simulink model "Part1_planarBicopter"  (R2020b)
settings: Solver=ode1  StartTime=0.0  StopTime=100  FixedStep=0.001  RelTol=1e-3
undefined symbols (not defined in the file or in its folder): Kd_alt, Kd_pos, Kd_roll, Kp_alt, Kp_pos, Kp_roll, noise, u_star, variaciones, wind, x_star
libraries: commchan3 x3
settings Model: Creator=rushik  LastModifiedBy=da_co
settings DataIOCC: SaveState=on

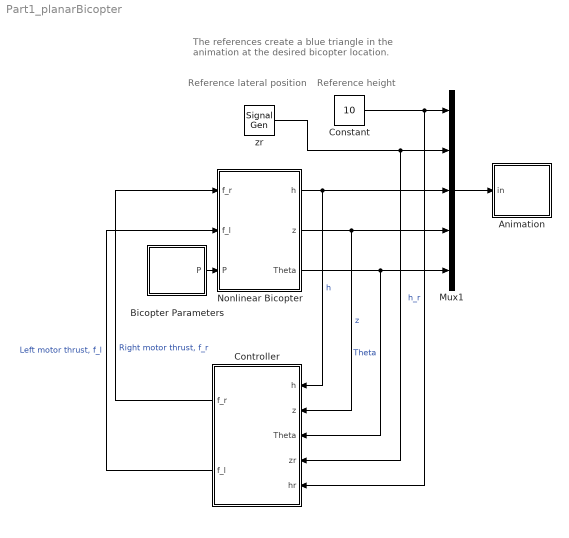
== system Part1_planarBicopter ==
  note: The references create a blue triangle in the
      | animation at the desired bicopter location.
  note: Reference height
  note: Reference lateral position
  Animation : Subsystem  mask(Pendulum plot){}
      mask help: Pendulum plot
      mask Help: Pendulum animation function using Handle graphics.
      mask Display: plot([-2 2],[10 10],[-2.5 -1.5],[10.5 10.5],[1.5 2.5],[10.5 10.5],0,0,0,20)
  Bicopter Parameters : Subsystem  mask{M=1, mRotor=0.25, J=0.0042, d=0.3, mu=0.1, g=9.81, x0=[0;0;0;0;0;0], noVar=noise, vWind=wind, distPercent=variaciones}
      mask prompts: M "Hub Mass"; mRotor "Motor Propeller Mass"; J "Hub Inertia"; d "Arm Length"; mu "Momentum Drag Coefficient"; g "Gravity"; x0 "Initial State"; noVar "Noise Variance"; vWind "Wind Velocity"; distPercent "Parameter Variation Percentage"
      mask TypeOptions M: Constant1/Value
      mask TypeOptions mRotor: Constant2/Value
      mask TypeOptions J: Constant3/Value
      mask TypeOptions d: Constant4/Value
      mask TypeOptions mu: Constant5/Value
      mask TypeOptions g: Constant6/Value
      mask TypeOptions x0: Constant7/Value
      mask TypeOptions noVar: Constant8/Value
      mask TypeOptions vWind: Constant10/Value
      mask TypeOptions distPercent: Constant9/Value
  Constant : Constant  Value=10
  Controller : Subsystem
  Mux1 : Mux  Inputs=5
  Nonlinear Bicopter : Subsystem
  zr : SignalGenerator  WaveForm=square  Amplitude=1.5  Frequency=0.05
  wires:
  Nonlinear Bicopter/1(h) -> Controller/1(h), Mux1/3  "h"
  Nonlinear Bicopter/2(z) -> Mux1/4, Controller/2(z)  "z"
  Nonlinear Bicopter/3(Theta) -> Mux1/5, Controller/3(Theta)  "Theta"
  Mux1/1 -> Animation/1(in)
  Bicopter Parameters/1(P) -> Nonlinear Bicopter/3(P)
  Controller/1(f_r) -> Nonlinear Bicopter/1(f_r)  "Right motor thrust, f_r"
  Controller/2(f_l) -> Nonlinear Bicopter/2(f_l)  "Left motor thrust, f_l"
  Constant/1 -> Controller/5(hr), Mux1/1  "h_r"
  zr/1 -> Controller/4(zr), Mux1/2

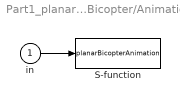
== system Part1_planarBicopter/Animation ==
  in : Inport
  S-function : S-Function  FunctionName=planarBicopterAnimation  SFunctionDeploymentMode=off  EnableBusSupport=off
      settings: DeleteFcn=pendan([],[],[],'DeleteBlock');
  wires:
  in/1 -> S-function/1

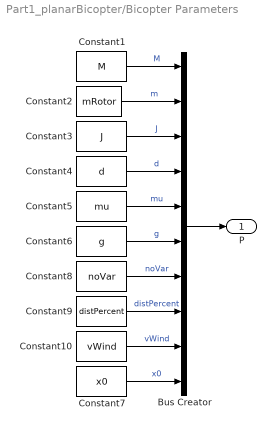
== system Part1_planarBicopter/Bicopter Parameters ==
  Bus Creator : BusCreator  Inputs=10
  Constant1 : Constant  Value=M
  Constant10 : Constant  Value=vWind  VectorParams1D=off
  Constant2 : Constant  Value=mRotor
  Constant3 : Constant  Value=J
  Constant4 : Constant  Value=d
  Constant5 : Constant  Value=mu
  Constant6 : Constant  Value=g
  Constant7 : Constant  Value=x0  VectorParams1D=off
  Constant8 : Constant  Value=noVar  VectorParams1D=off
  Constant9 : Constant  Value=distPercent  VectorParams1D=off
  P : Outport
  wires:
  Bus Creator/1 -> P/1
  Constant7/1 -> Bus Creator/10  "x0"
  Constant5/1 -> Bus Creator/5  "mu"
  Constant3/1 -> Bus Creator/3  "J"
  Constant2/1 -> Bus Creator/2  "m"
  Constant6/1 -> Bus Creator/6  "g"
  Constant4/1 -> Bus Creator/4  "d"
  Constant1/1 -> Bus Creator/1  "M"
  Constant8/1 -> Bus Creator/7  "noVar"
  Constant9/1 -> Bus Creator/8  "distPercent"
  Constant10/1 -> Bus Creator/9  "vWind"

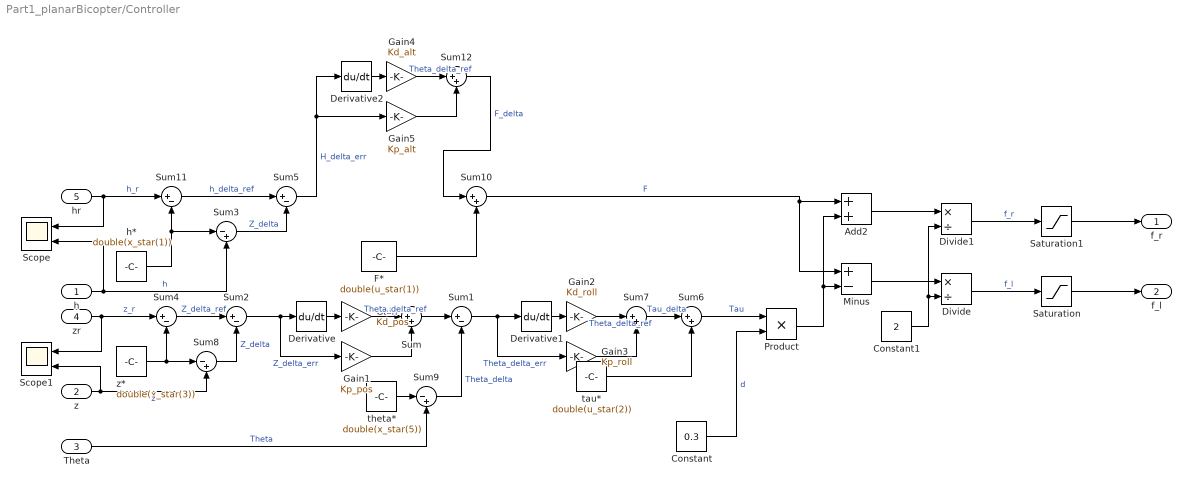
== system Part1_planarBicopter/Controller ==
  h : Inport
  z : Inport  Port=2
  Theta : Inport  Port=3
  zr : Inport  Port=4
  hr : Inport  Port=5
  Add2 : Sum
  Constant : Constant  Value=0.3
  Constant1 : Constant  Value=2
  Derivative : Derivative
  Derivative1 : Derivative
  Derivative2 : Derivative
  Divide : Product  Inputs=*/
  Divide1 : Product  Inputs=*/
  F* : Constant  Value=double(u_star(1))
  Gain : Gain  Gain=Kd_pos
  Gain1 : Gain  Gain=Kp_pos
  Gain2 : Gain  Gain=Kd_roll
  Gain3 : Gain  Gain=Kp_roll
  Gain4 : Gain  Gain=Kd_alt
  Gain5 : Gain  Gain=Kp_alt
  Minus : Sum  Inputs=+-
  Product : Product
  Saturation : Saturate  UpperLimit=10  LowerLimit=0
  Saturation1 : Saturate  UpperLimit=10  LowerLimit=0
  Scope : Scope  NumInputPorts=2
  Scope1 : Scope  NumInputPorts=2
  Sum{,6..7,10,12} (5 alike) : Sum  Inputs=|++
  Sum{1..2,4..5,11} (5 alike) : Sum  Inputs=|+-
  Sum3 : Sum  Inputs=|-+
  Sum8 : Sum  Inputs=|-+
  Sum9 : Sum  Inputs=|-+
  h* : Constant  Value=double(x_star(1))
  tau* : Constant  Value=double(u_star(2))
  theta* : Constant  Value=double(x_star(5))
  z* : Constant  Value=double(x_star(3))
  f_r : Outport
  f_l : Outport  Port=2
  wires:
  z/1 -> Scope1/2, Sum8/2  "z"
  Theta/1 -> Sum9/2  "Theta"
  zr/1 -> Sum4/1, Scope1/1  "z_r"
  Gain/1 -> Sum/1  "Theta_delta_ref"
  h/1 -> Scope/2, Sum3/2  "h"
  Minus/1 -> Divide/1
  Product/1 -> Minus/2, Add2/2
  Constant/1 -> Product/2  "d"
  Constant1/1 -> Divide1/2, Divide/2
  Add2/1 -> Divide1/1
  Sum10/1 -> Add2/1, Minus/1  "F"
  F*/1 -> Sum10/2
  Sum1/1 -> Gain3/1, Derivative1/1  "Theta_delta_err"
  Divide1/1 -> Saturation1/1  "f_r"
  Saturation1/1 -> f_r/1
  Divide/1 -> Saturation/1  "f_l"
  Saturation/1 -> f_l/1
  Sum12/1 -> Sum10/1  "F_delta"
  Sum2/1 -> Gain1/1, Derivative/1  "Z_delta_err"
  hr/1 -> Sum11/1, Scope/1  "h_r"
  Sum4/1 -> Sum2/1  "Z_delta_ref"
  z*/1 -> Sum8/1, Sum4/2
  theta*/1 -> Sum9/1
  Sum7/1 -> Sum6/1  "Tau_delta"
  tau*/1 -> Sum6/2
  Sum6/1 -> Product/1  "Tau"
  Sum8/1 -> Sum2/2  "Z_delta"
  Sum9/1 -> Sum1/2  "Theta_delta"
  Sum11/1 -> Sum5/1  "h_delta_ref"
  h*/1 -> Sum3/1, Sum11/2
  Sum3/1 -> Sum5/2  "Z_delta"
  Sum5/1 -> Gain5/1, Derivative2/1  "H_delta_err"
  Derivative/1 -> Gain/1
  Sum/1 -> Sum1/1
  Gain1/1 -> Sum/2
  Derivative1/1 -> Gain2/1
  Gain2/1 -> Sum7/1  "Theta_delta_ref"
  Gain3/1 -> Sum7/2
  Derivative2/1 -> Gain4/1
  Gain4/1 -> Sum12/1  "Theta_delta_ref"
  Gain5/1 -> Sum12/2

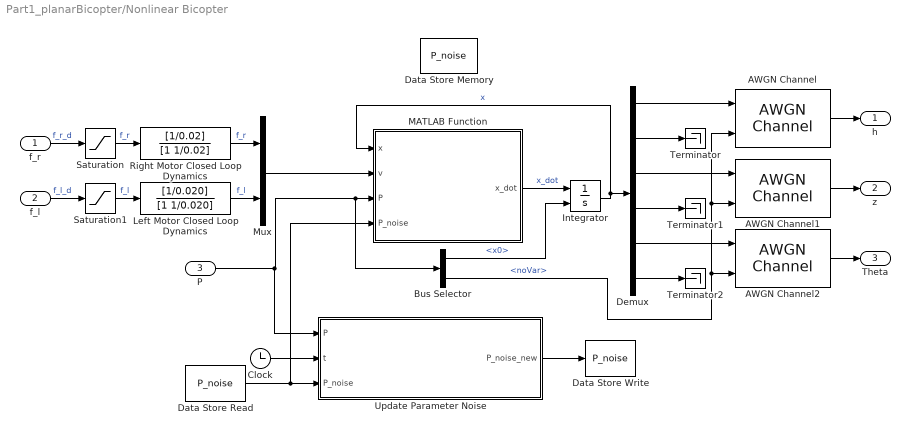
== system Part1_planarBicopter/Nonlinear Bicopter ==
  f_r : Inport
  f_l : Inport  Port=2
  P : Inport  Port=3
  AWGN Channel : commchan3/AWGN Channel  InputProcessing=Columns as channels (frame based)  seed=67  noiseMode=Variance from port  EbNodB=10  EsNodB=10  SNRdB=10  bitsPerSym=1  Ps=1  Tsym=1  variance=1
  AWGN Channel1 : commchan3/AWGN Channel  InputProcessing=Columns as channels (frame based)  seed=67  noiseMode=Variance from port  EbNodB=10  EsNodB=10  SNRdB=10  bitsPerSym=1  Ps=1  Tsym=1  variance=1
  AWGN Channel2 : commchan3/AWGN Channel  InputProcessing=Columns as channels (frame based)  seed=67  noiseMode=Variance from port  EbNodB=10  EsNodB=10  SNRdB=10  bitsPerSym=1  Ps=1  Tsym=1  variance=1
  Bus Selector : BusSelector  OutputSignals=x0,noVar
  Clock : Clock
  Data Store Memory : DataStoreMemory  DataStoreName=P_noise  ReadBeforeWriteMsg=warning  WriteAfterWriteMsg=warning  WriteAfterReadMsg=warning  InitialValue=[0;0;0;0;0;0;0;0]  ShowAdditionalParam=off  OutDataTypeStr=double
  Data Store Read : DataStoreRead  DataStoreName=P_noise
  Data Store Write : DataStoreWrite  DataStoreName=P_noise
  Demux : Demux  Outputs=6
  Integrator : Integrator  InitialConditionSource=external
  Left Motor Closed Loop Dynamics : TransferFcn  Numerator=[1/0.020]  Denominator=[1 1/0.020]
  MATLAB Function : MATLAB Function  TreatAsAtomicUnit=on
  Mux : Mux  Inputs=2
  Right Motor Closed Loop Dynamics : TransferFcn  Numerator=[1/0.02]  Denominator=[1 1/0.02]
  Saturation : Saturate  UpperLimit=[10]  LowerLimit=[0]  ZeroCross=off
  Saturation1 : Saturate  UpperLimit=[10]  LowerLimit=[0]  ZeroCross=off
  Terminator : Terminator
  Terminator1 : Terminator
  Terminator2 : Terminator
  Update Parameter Noise : MATLAB Function  TreatAsAtomicUnit=on
  h : Outport
  z : Outport  Port=2
  Theta : Outport  Port=3
  wires:
  MATLAB Function/1(x_dot) -> Integrator/1  "x_dot"
  f_r/1 -> Saturation/1  "f_r_d"
  Bus Selector/1 -> Integrator/2  "<x0>"
  P/1 -> Update Parameter Noise/1(P), Bus Selector/1, MATLAB Function/3(P)
  f_l/1 -> Saturation1/1  "f_l_d"
  Demux/6 -> Terminator2/1
  Demux/2 -> Terminator/1
  Demux/4 -> Terminator1/1
  Integrator/1 -> MATLAB Function/1(x), Demux/1  "x"
  Bus Selector/2 -> AWGN Channel2/2, AWGN Channel1/2, AWGN Channel/2  "<noVar>"
  Demux/1 -> AWGN Channel/1
  Demux/3 -> AWGN Channel1/1
  Demux/5 -> AWGN Channel2/1
  AWGN Channel/1 -> h/1
  AWGN Channel1/1 -> z/1
  AWGN Channel2/1 -> Theta/1
  Update Parameter Noise/1(P_noise_new) -> Data Store Write/1
  Clock/1 -> Update Parameter Noise/2(t)
  Data Store Read/1 -> MATLAB Function/4(P_noise), Update Parameter Noise/3(P_noise)
  Mux/1 -> MATLAB Function/2(v)
  Saturation1/1 -> Left Motor Closed Loop Dynamics/1  "f_l"
  Saturation/1 -> Right Motor Closed Loop Dynamics/1  "f_r"
  Right Motor Closed Loop Dynamics/1 -> Mux/1  "f_r"
  Left Motor Closed Loop Dynamics/1 -> Mux/2  "f_l"

== matlab function Part1_planarBicopter/Nonlinear Bicopter/MATLAB Function ==
  settings: updateMethod=DISCRETE
  data: x input; v input; x_dot output; P input; P_noise input
function x_dot = VTOLNonlinearDynamics(x,v,P, P_noise)

M = P(1) + P_noise(1);
m = P(2) + P_noise(2);
J = P(3) + P_noise(3);
d = P(4) + P_noise(4);
mu = P(5)+ P_noise(5);
g = P(6) + P_noise(6);
c_d = 1;
v_wind = P(9) + P_noise(7);
theta_wind = P_noise(8);

F_drag_wind_vert = c_d*v_wind*sin(theta_wind);
F_drag_wind_horiz = c_d*v_wind*cos(theta_wind);

thrustToTorque = [1   1;
                  d  -d];

u = thrustToTorque*v;

h = x(1);
hD = x(2);
z = x(3);
zD = x(4);
T = x(5);
TD = x(6);

F = u(1);
tau = u(2);

x_dot = [hD;
         -g + (1/(M + 2*m)) * (cos(T) * F + F_drag_wind_vert);
         zD;
         (1/(M + 2*m)) * (-mu * zD - sin(T) * F + F_drag_wind_horiz);
         TD;
         (1/(2 * m * d^2 + J)) * tau];
     
end

== matlab function Part1_planarBicopter/Nonlinear Bicopter/Update Parameter Noise ==
  settings: updateMethod=DISCRETE
  data: P input; t input; P_noise_new output; P_noise input
function P_noise_new  = updateParameterNoise(P,t,P_noise)
if t<=0.001
    M = P(1) ;
    m = P(2) ;
    J = P(3) ;
    d = P(4) ;
    mu = P(5);
    g = P(6) ;
    distPercent = P(8);
    MNoise = (distPercent*M/100)*rand - distPercent*M/200;
    mNoise = (distPercent*m/100)*rand - distPercent*m/200;
    JNoise = (distPercent*J/100)*rand - distPercent*J/200;
    dNoise = (distPercent*d/100)*rand - distPercent*d/200;
    muNoise = (distPercent*mu/100)*rand - distPercent*mu/200;
    gNoise = (distPercent*g/100)*rand - distPercent*g/200;
    
    P_noise_new = ...
    [MNoise ;
     mNoise ;
     JNoise ;
     dNoise ;
    muNoise ;
     gNoise;
     P_noise(7);
     P_noise(8)];
elseif mod(round(t/0.002),1000)==0 %0.002 is the sample time
    vWind = P(9);
    vWindNoise = 20*vWind/100*rand - 20*vWind/200;
    thetaWindNoise = (0.5)*rand - 0.25;
    P_noise_new = ...
    [P_noise(1:6,1);
     vWindNoise;
     thetaWindNoise];
else
    P_noise_new = P_noise;
end
